simulink model "flightController"  (R2023b)
settings: Solver=ode3  StartTime=0  StopTime=TFinal  FixedStep=Ts  RelTol=1e-3  EnableMultiTasking=on
undefined symbols (not defined in the file): Controller, DiscIntNeverNeededParam, g, PD, PI, PID, Ts, Vehicle
libraries: simulink x7, slpidlib x3, rllib x2, dspstat3 x2, fuzblock x2
(part 1 of 2)
settings Model: Creator=The MathWorks, Inc.  LastModifiedBy=mrkaplan
settings SolverCC: AlgebraicLoopSolver=TrustRegion  MinimalZcImpactIntegration=on
settings DataIOCC: LimitDataPoints=on  SaveFormat=Array  ReturnWorkspaceOutputs=off
settings OptimizationCC: BlockReduction=off  DefaultParameterBehavior=Inlined  BufferReuse=off  PassReuseOutputArgsThreshold=0
settings DebuggingCC: AlgebraicLoopMsg=none  MultiTaskRateTransMsg=warning  ParameterPrecisionLossMsg=none  ParameterTunabilityLossMsg=error  BusObjectLabelMismatch=error  SFUnexpectedBacktrackingDiag=warning  SFNoUnconditionalDefaultTransitionDiag=warning  SFExecutionAtInitializationDiag=none  ArithmeticOperatorsInVariantConditions=warning
settings HardwareCC: ProdBitPerPointer=32  ProdBitPerSizeT=32  ProdBitPerPtrDiffT=32  ProdLargestAtomicInteger=Long  ProdWordSize=32  ProdHWDeviceType=ARM Compatible->ARM 9
settings ModelReferenceCC: EnableRefExpFcnMdlSchedulingChecks=on  ModelReferenceNumInstancesAllowed=Single  PropagateSignalLabelsOutOfModel=off
settings SFSimCC: SimUseLocalCustomCode=off  CustomCodeUndefinedFunction=UseInterfaceOnly
settings RTWCC: GenerateReport=on  RTWUseLocalCustomCode=off  LaunchReport=on
settings CodeAppCC: ForceParamTrailComments=on  MaxIdLength=63  OperatorAnnotations=on  StateflowObjectComments=on  MATLABSourceComments=on
settings GRTTargetCC: TargetLangStandard=C89/C90 (ANSI)
settings ConfigComp: CovMetricSettings=dw  CovSaveCumulativeToWorkspaceVar=on  CovSaveSingleToWorkspaceVar=on  CovExternalEMLEnable=off  CovSFcnEnable=off

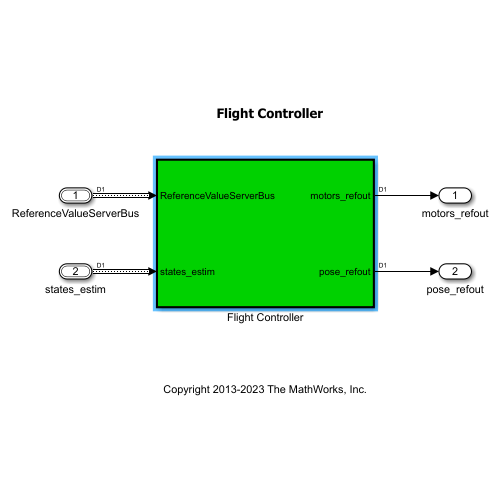
[thumbnail: Simulink's stored preview of the top-level diagram]
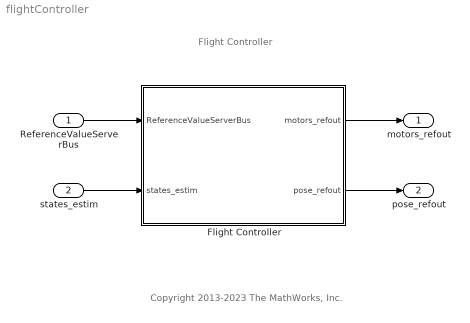
== system flightController ==
  note: Flight Controller
  note: Copyright 2013-2023 The MathWorks, Inc.
  ReferenceValueServerBus : Inport  OutDataTypeStr=Bus: CommandBus  BusOutputAsStruct=on
  states_estim : Inport  Port=2  OutDataTypeStr=Bus: statesEstim_t  BusOutputAsStruct=on
  Flight Controller : Subsystem  TreatAsAtomicUnit=on
  motors_refout : Outport  VectorParamsAs1DForOutWhenUnconnected=off
  pose_refout : Outport  Port=2  VectorParamsAs1DForOutWhenUnconnected=off
  wires:
  ReferenceValueServerBus/1 -> Flight Controller/1(ReferenceValueServerBus)
  states_estim/1 -> Flight Controller/2(states_estim)
  Flight Controller/2(pose_refout) -> pose_refout/1
  Flight Controller/1(motors_refout) -> motors_refout/1

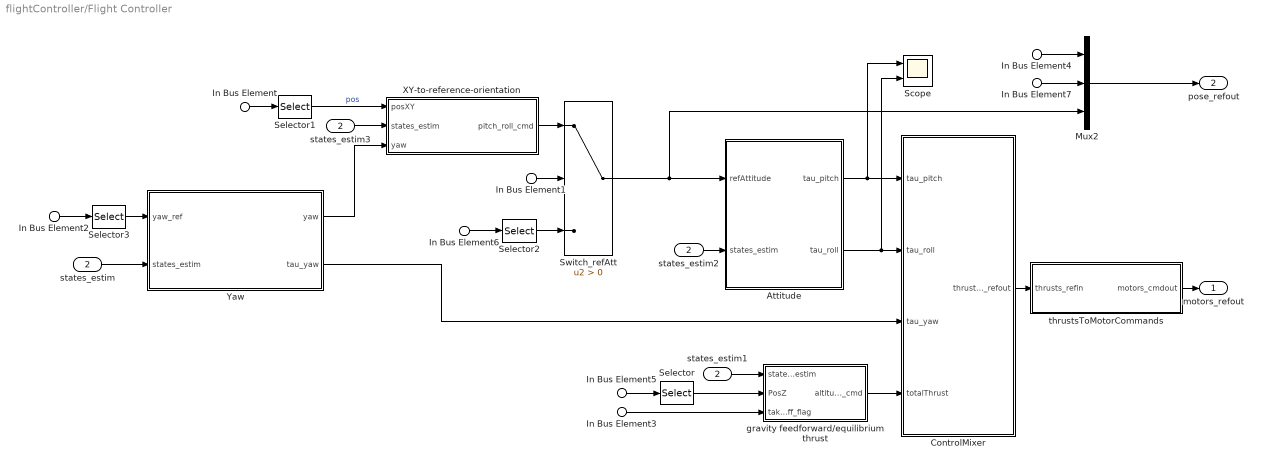
== system flightController/Flight Controller ==
  In Bus Element1 : Inport  PortName=ReferenceValueServerBus  Element=controlModePosVSOrient
  In Bus Element : Inport  PortName=ReferenceValueServerBus  Element=pos_ref
  In Bus Element4 : Inport  PortName=ReferenceValueServerBus  Element=pos_ref
  In Bus Element5 : Inport  PortName=ReferenceValueServerBus  Element=pos_ref
  In Bus Element2 : Inport  PortName=ReferenceValueServerBus  Element=orient_ref
  In Bus Element6 : Inport  PortName=ReferenceValueServerBus  Element=orient_ref
  In Bus Element7 : Inport  PortName=ReferenceValueServerBus  Element=orient_ref
  In Bus Element3 : Inport  PortName=ReferenceValueServerBus  Element=takeoff_flag
  states_estim : Inport  Port=2
  Attitude : Subsystem  Variant=on  VariantControlMode=label  VariantControl=Attitude  LabelModeActiveChoice=RL
  ControlMixer : Subsystem
  Mux2 : Mux  Inputs=3
  Scope : Scope  NumInputPorts=2
  Selector : Selector  InputPortWidth=3  IndexOptions=Index vector (dialog)  Indices=3  OutputSizes=1
  Selector1 : Selector  InputPortWidth=3  IndexOptions=Index vector (dialog)  Indices=[1 2]  OutputSizes=1
  Selector2 : Selector  InputPortWidth=3  IndexOptions=Index vector (dialog)  Indices=[2 3]  OutputSizes=1
  Selector3 : Selector  InputPortWidth=3  IndexOptions=Index vector (dialog)  Indices=1  OutputSizes=1
  Switch_refAtt : Switch  Criteria=u2 > Threshold  SaturateOnIntegerOverflow=off  InputSameDT=off
  XY-to-reference-orientation : Subsystem
  Yaw : Subsystem  Variant=on  VariantControlMode=label  VariantControl=Yaw  LabelModeActiveChoice=PD
  gravity feedforward/equilibrium thrust : Subsystem
  states_estim1 : InportShadow  Port=2
  states_estim2 : InportShadow  Port=2
  states_estim3 : InportShadow  Port=2
  thrustsToMotorCommands : Subsystem
  motors_refout : Outport  VectorParamsAs1DForOutWhenUnconnected=off
  pose_refout : Outport  Port=2  VectorParamsAs1DForOutWhenUnconnected=off
  wires:
  thrustsToMotorCommands/1(motors_cmdout) -> motors_refout/1
  In Bus Element1/1 -> Switch_refAtt/2
  XY-to-reference-orientation/1(pitch_roll_cmd) -> Switch_refAtt/1
  In Bus Element2/1 -> Selector3/1
  In Bus Element/1 -> Selector1/1
  Selector1/1 -> XY-to-reference-orientation/1(posXY)  "pos"
  ControlMixer/1(thrusts_refout) -> thrustsToMotorCommands/1(thrusts_refin)
  In Bus Element3/1 -> gravity feedforward/equilibrium thrust/3(takeoff_flag)
  Switch_refAtt/1 -> Mux2/3, Attitude/1(refAttitude)
  gravity feedforward/equilibrium thrust/1(altitude_cmd) -> ControlMixer/4(totalThrust)
  Mux2/1 -> pose_refout/1
  states_estim1/1 -> gravity feedforward/equilibrium thrust/1(states_estim)
  states_estim3/1 -> XY-to-reference-orientation/2(states_estim)
  In Bus Element4/1 -> Mux2/1
  Selector/1 -> gravity feedforward/equilibrium thrust/2(PosZ)
  In Bus Element5/1 -> Selector/1
  In Bus Element6/1 -> Selector2/1
  Selector2/1 -> Switch_refAtt/3
  In Bus Element7/1 -> Mux2/2
  states_estim2/1 -> Attitude/2(states_estim)
  Attitude/1(tau_pitch) -> Scope/1, ControlMixer/1(tau_pitch)
  Attitude/2(tau_roll) -> Scope/2, ControlMixer/2(tau_roll)
  Selector3/1 -> Yaw/1(yaw_ref)
  states_estim/1 -> Yaw/2(states_estim)
  Yaw/1(yaw) -> XY-to-reference-orientation/3(yaw)
  Yaw/2(tau_yaw) -> ControlMixer/3(tau_yaw)

== system flightController/Flight Controller/Attitude ==
  refAttitude : Inport
  states_estim : Inport  Port=2
  Roll & Pitch PID Controller : Subsystem  VariantControl=PID
  Roll & Pitch RL Agent : Subsystem  VariantControl=RL
  Roll & Pitch RL Based PID Controller : Subsystem  VariantControl=RL Based PID
  tau_pitch : Outport
  tau_roll : Outport  Port=2

== system flightController/Flight Controller/ControlMixer ==
  tau_pitch : Inport
  tau_roll : Inport  Port=2
  tau_yaw : Inport  Port=3
  totalThrust : Inport  Port=4
  Mux2 : Mux
  Product : Product  Multiplication=Matrix(*)  RndMeth=Zero
  TorqueTotalThrustToThrustPerMotor : Constant  Value=Controller.Q2Ts  OutDataTypeStr=single
  thrusts_refout : Outport  VectorParamsAs1DForOutWhenUnconnected=off
  wires:
  Product/1 -> thrusts_refout/1
  tau_roll/1 -> Mux2/4
  tau_pitch/1 -> Mux2/3
  tau_yaw/1 -> Mux2/2
  totalThrust/1 -> Mux2/1
  TorqueTotalThrustToThrustPerMotor/1 -> Product/1
  Mux2/1 -> Product/2

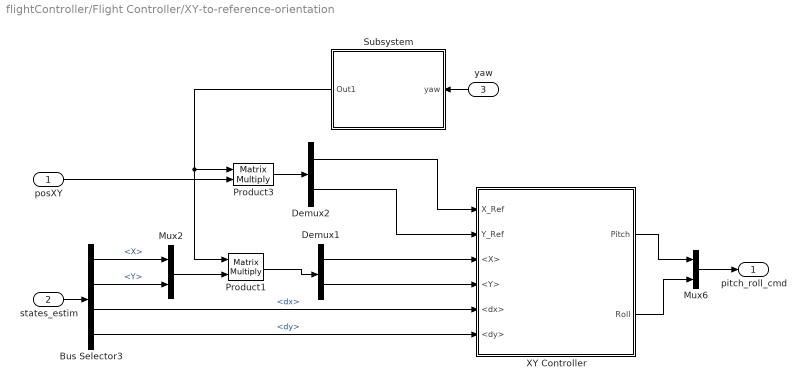
== system flightController/Flight Controller/XY-to-reference-orientation ==
  posXY : Inport
  states_estim : Inport  Port=2
  yaw : Inport  Port=3
  Bus Selector3 : BusSelector  OutputSignals=X,Y,dx,dy
  Demux1 : Demux  Outputs=2
  Demux2 : Demux  Outputs=2
  Mux2 : Mux  Inputs=2
  Mux6 : Mux  Inputs=2
  Product1 : Product  Multiplication=Matrix(*)  OutDataTypeStr=single  RndMeth=Zero
  Product3 : Product  Multiplication=Matrix(*)  OutDataTypeStr=single  RndMeth=Zero
  Subsystem : Subsystem
  "XY Controller " : Subsystem  Variant=on  VariantControlMode=label  VariantControl=Variant2  LabelModeActiveChoice=PD
  pitch_roll_cmd : Outport  VectorParamsAs1DForOutWhenUnconnected=off
  wires:
  Mux6/1 -> pitch_roll_cmd/1
  Demux1/2 -> "XY Controller "/4("<Y> ")
  posXY/1 -> Product3/2
  Demux2/2 -> "XY Controller "/2(Y_Ref)
  Subsystem/1(Out1) -> Product3/1, Product1/1
  Demux2/1 -> "XY Controller "/1(X_Ref)
  states_estim/1 -> Bus Selector3/1
  Demux1/1 -> "XY Controller "/3("<X> ")
  Mux2/1 -> Product1/2
  yaw/1 -> Subsystem/1(yaw)
  Product1/1 -> Demux1/1
  Bus Selector3/3 -> "XY Controller "/5("<dx> ")  "<dx>"
  Bus Selector3/4 -> "XY Controller "/6("<dy> ")  "<dy>"
  Bus Selector3/2 -> Mux2/2  "<Y>"
  Bus Selector3/1 -> Mux2/1  "<X>"
  Product3/1 -> Demux2/1
  "XY Controller "/1(" Pitch") -> Mux6/1
  "XY Controller "/2(" Roll") -> Mux6/2

== system flightController/Flight Controller/Yaw ==
  yaw_ref : Inport
  states_estim : Inport  Port=2
  Yaw PD Controller : Subsystem  VariantControl=PD
  Yaw RL Agent : Subsystem  VariantControl=RL
  yaw : Outport
  tau_yaw : Outport  Port=2

== system flightController/Flight Controller/gravity feedforward//equilibrium thrust ==
  note: ALTITUDE
  states_estim : Inport
  PosZ : Inport  Port=2
  takeoff_flag : Inport  Port=3
  Bus Selector6 : BusSelector  OutputSignals=Z,dz
  SaturationThrust : Saturate  UpperLimit=4*Controller.totalThrustMaxRelative*Controller.motorsThrustPerMotorMax  LowerLimit=-4*Controller.totalThrustMaxRelative*Controller.motorsThrustPerMotorMax  OutDataTypeStr=single
  Sum4 : Sum  Inputs=++|  OutDataTypeStr=single  AccumDataTypeStr=single  SaturateOnIntegerOverflow=on
  TakeoffOrControl_Switch : Switch  Criteria=u2 > Threshold  SaturateOnIntegerOverflow=off  InputSameDT=off
  Z Controller Subsystem : Subsystem  Variant=on  VariantControlMode=label  VariantControl=Variant2  LabelModeActiveChoice=PD
  takeoff_gain : Gain  Gain=Controller.takeoffGain  ParamDataTypeStr=single  OutDataTypeStr=single  SaturateOnIntegerOverflow=on
  w0 : Constant  Value=-g*Vehicle.Airframe.mass  OutDataTypeStr=single  SampleTime=Ts
  altitude_cmd : Outport  VectorParamsAs1DForOutWhenUnconnected=off
  wires:
  Z Controller Subsystem/1(" Altitude") -> TakeoffOrControl_Switch/3
  takeoff_flag/1 -> TakeoffOrControl_Switch/2
  PosZ/1 -> Z Controller Subsystem/1("PosZ ")
  states_estim/1 -> Bus Selector6/1
  takeoff_gain/1 -> TakeoffOrControl_Switch/1
  Sum4/1 -> SaturationThrust/1
  w0/1 -> Sum4/1, takeoff_gain/1
  Bus Selector6/2 -> Z Controller Subsystem/3("<dz> ")  "<dz>"
  SaturationThrust/1 -> altitude_cmd/1
  Bus Selector6/1 -> Z Controller Subsystem/2("<Z> ")  "<Z>"
  TakeoffOrControl_Switch/1 -> Sum4/2

== system flightController/Flight Controller/thrustsToMotorCommands ==
  thrusts_refin : Inport
  MotorDirections : Gain  Gain=[1 -1 1 -1]
  Saturation5 : Saturate  UpperLimit=Vehicle.Motor.maxLimit  LowerLimit=Vehicle.Motor.minLimit
  ThrustToMotorCommand : Gain  Gain=-Vehicle.Motor.thrustToMotorCommand
  motors_cmdout : Outport  VectorParamsAs1DForOutWhenUnconnected=off
  wires:
  Saturation5/1 -> MotorDirections/1
  MotorDirections/1 -> motors_cmdout/1
  ThrustToMotorCommand/1 -> Saturation5/1
  thrusts_refin/1 -> ThrustToMotorCommand/1

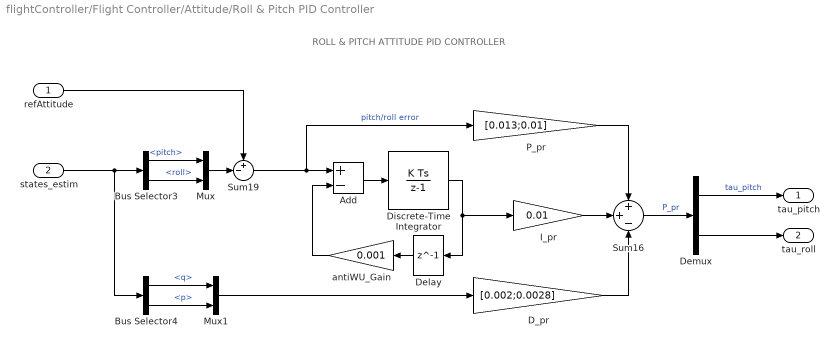
== system flightController/Flight Controller/Attitude/Roll & Pitch PID Controller ==
  note: ROLL & PITCH ATTITUDE PID CONTROLLER
  refAttitude : Inport
  states_estim : Inport  Port=2
  Add : Sum  Inputs=+-
  Bus Selector3 : BusSelector  OutputSignals=pitch,roll
  Bus Selector4 : BusSelector  OutputSignals=q,p
  D_pr : Gain  Gain=[0.002;0.0028]
  Delay : Delay  DelayLength=1  InitialCondition=0
  Demux : Demux  Outputs=2
  Discrete-Time Integrator : DiscreteIntegrator  SampleTime=Ts  LimitOutput=on  UpperSaturationLimit=2  LowerSaturationLimit=-2  ICPrevOutput=DiscIntNeverNeededParam  ICPrevScaledInput=DiscIntNeverNeededParam
  I_pr : Gain  Gain=0.01
  Mux : Mux  Inputs=2
  Mux1 : Mux  Inputs=2
  P_pr : Gain  Gain=[0.013;0.01]
  Sum16 : Sum  Inputs=++-  OutDataTypeStr=single  AccumDataTypeStr=single  SaturateOnIntegerOverflow=on
  Sum19 : Sum  Inputs=+-|
  antiWU_Gain : Gain  Gain=0.001
  tau_pitch : Outport  VectorParamsAs1DForOutWhenUnconnected=off
  tau_roll : Outport  Port=2  VectorParamsAs1DForOutWhenUnconnected=off
  wires:
  Sum16/1 -> Demux/1  "P_pr"
  antiWU_Gain/1 -> Add/2
  Add/1 -> Discrete-Time Integrator/1
  Bus Selector3/1 -> Mux/1  "<pitch>"
  Bus Selector4/1 -> Mux1/1  "<q>"
  P_pr/1 -> Sum16/1
  I_pr/1 -> Sum16/2
  Sum19/1 -> Add/1, P_pr/1  "pitch/roll error"
  Discrete-Time Integrator/1 -> Delay/1, I_pr/1
  Delay/1 -> antiWU_Gain/1
  Demux/1 -> tau_pitch/1  "tau_pitch"
  Demux/2 -> tau_roll/1
  D_pr/1 -> Sum16/3
  states_estim/1 -> Bus Selector3/1, Bus Selector4/1
  refAttitude/1 -> Sum19/1
  Mux/1 -> Sum19/2
  Bus Selector3/2 -> Mux/2  "<roll>"
  Mux1/1 -> D_pr/1
  Bus Selector4/2 -> Mux1/2  "<p>"

== system flightController/Flight Controller/Attitude/Roll & Pitch RL Agent ==
  note: RL BASED ROLL & PITCH ATTITUDE CONTROLLER
  refAttitude : Inport
  states_estim : Inport  Port=2
  Data Type Conversion : DataTypeConversion  OutDataTypeStr=single  SaturateOnIntegerOverflow=off  RndMeth=Floor
  Demux : Demux  Outputs=2
  Display : Display
  RL Agent : rllib/RL Agent  Agent=PPOagentObj  ExternalActionAsInput=off  ProvideLastAction=off  ProvideCumRwd=on  TreatAsDirectFeedthrough=on  UseStrictObservationDataTypes=off
  Saturation : Saturate  UpperLimit=0.005  LowerLimit=-0.005
  Saturation1 : Saturate  UpperLimit=0.005  LowerLimit=-0.005
  Unit Delay : UnitDelay  SampleTime=-1  HasFrameUpgradeWarning=on
  observations : Subsystem
  rewardFunction : Subsystem
      settings: PortSchema="{\"entries\":[{\"content\":{\"sides\":[{\"content\":{\"connectorIds\":[\"In1\",\"In2\"]},\"type\":\"ConnectorPlacement.EquallySpacedRectSide\",\"uuid\":\"a67b2643-6d4e-47da-9384-3a1e9a412811\"},{\"content\":{\"connectorIds\":[\"Out1\",\"Out2\"],\"side\":\"RIGHT\"},\"type\":\"ConnectorPlacement.EquallySpacedRectSide\",\"uuid\":\"5cf99017-b414-4804-a368-110af44f7389\"},{\"content\":{\"connectorIds\":[\"In3\"],\"side\":\"TOP\"},\"type\":\"ConnectorPlacement.EquallySpacedRectSide\",\"uuid\":\"c082dbf4-38c8-469f-94b4-9bfadc9c0830\"}]},\"type\":\"ConnectorPlacement.EquallySpacedConnector\",\"uuid\":\"aea0a46f-4b15-48f6-a1a1-f72f4d47f5c8\"}],\"packageUris\":[\"http://schema.mathworks.com/mf0/Connector/R2020b\"],\"version\":\"1.0\"}"
  tau_pitch : Outport  VectorParamsAs1DForOutWhenUnconnected=off
  tau_roll : Outport  Port=2  VectorParamsAs1DForOutWhenUnconnected=off
  wires:
  rewardFunction/1(Out1) -> RL Agent/2
  refAttitude/1 -> observations/1(refAttitude), rewardFunction/1(In2)
  states_estim/1 -> observations/2(states_estim), rewardFunction/2(In1)
  Demux/2 -> Saturation1/1  "tau_roll"
  Demux/1 -> Saturation/1  "tau_pitch"
  RL Agent/1 -> Unit Delay/1, Data Type Conversion/1
  Data Type Conversion/1 -> Demux/1
  observations/1(Out1) -> RL Agent/1
  rewardFunction/2(Out2) -> RL Agent/3
  Saturation/1 -> tau_pitch/1
  Saturation1/1 -> tau_roll/1
  RL Agent/2 -> Display/1
  Unit Delay/1 -> rewardFunction/3(In3)

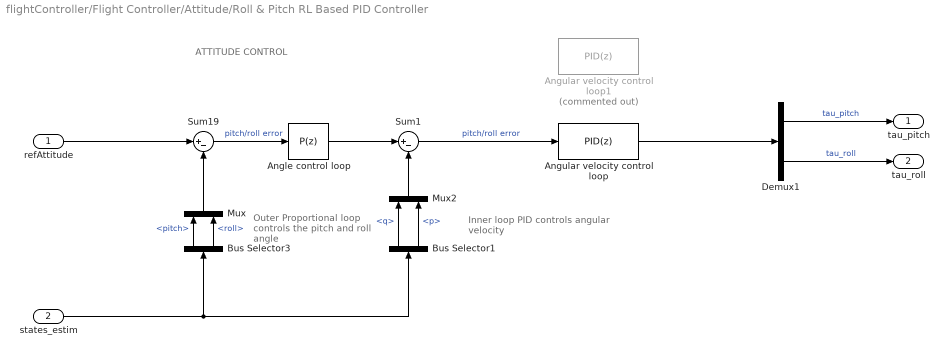
== system flightController/Flight Controller/Attitude/Roll & Pitch RL Based PID Controller ==
  note: ATTITUDE CONTROL
  note: Inner loop PID
      | controls angular velocity
  note: Outer Proportional loop
      | controls the pitch and roll angle
  refAttitude : Inport
  states_estim : Inport  Port=2
  Angle control loop : slpidlib/PID Controller  Controller=P  Form=Parallel  TimeDomain=Discrete-time  UseExternalTs=off  SampleTime=Ts  IntegratorMethod=Forward Euler  FilterMethod=Forward Euler  ControllerParametersSource=internal  P=4  I=1  UseKiTs=off  D=0  N=100  UseFilter=on  TunerSelectOption=Transfer Function Based (PID Tuner App)  InitialConditionSource=internal  InitialConditionForIntegrator=0  InitialConditionForFilter=0  DifferentiatorICPrevScaledInput=0  ExternalReset=none  TrackingMode=off  Kt=1  LimitOutput=off  SatLimitsSource=internal  UpperSaturationLimit=inf  LowerSaturationLimit=-inf  LinearizeAsGain=on  AntiWindupMode=none  Kb=1  LimitIntegrator=off  UpperIntegratorSaturationLimit=inf  LowerIntegratorSaturationLimit=-inf  POutMin=[]  POutMax=[]  IOutMin=[]  IOutMax=[]  DOutMin=[]  DOutMax=[]  NOutMin=[]  NOutMax=[]  SumOutMin=[]  SumOutMax=[]  SaturationOutMin=[]  SaturationOutMax=[]  PParamMin=[]  PParamMax=[]  IParamMin=[]  IParamMax=[]  DParamMin=[]  DParamMax=[]  NParamMin=[]  NParamMax=[]  KbParamMin=[]  KbParamMax=[]  KtParamMin=[]  KtParamMax=[]  KbOutMin=[]  KbOutMax=[]  KtOutMin=[]  KtOutMax=[]  IntegratorOutMin=[]  IntegratorOutMax=[]  FilterOutMin=[]  FilterOutMax=[]  SumI1OutMin=[]  SumI1OutMax=[]  SumI2OutMin=[]  SumI2OutMax=[]  SumI3OutMin=[]  SumI3OutMax=[]  SumI4OutMin=[]  SumI4OutMax=[]  SumDOutMin=[]  SumDOutMax=[]  DifferentiatorOutMin=[]  DifferentiatorOutMax=[]  FilterDiffOutCoefMin=[]  FilterDiffOutCoefMax=[]  ReciprocalOutMin=[]  ReciprocalOutMax=[]  SumDenOutMin=[]  SumDenOutMax=[]  SumNumOutMin=[]  SumNumOutMax=[]  DivideOutMin=[]  DivideOutMax=[]  UdiffTsProdOutMin=[]  UdiffTsProdOutMax=[]  NTsProdOutMin=[]  NTsProdOutMax=[]  UintegralTsProdOutMin=[]  UintegralTsProdOutMax=[]  UngainTsProdOutMin=[]  UngainTsProdOutMax=[]  ClampingZeroOutDataTypeStr=Inherit: Inherit via back propagation  ClampingZeroOutMin=[]  ClampingZeroOutMax=[]  FilterDenConstantOutDataTypeStr=Inherit: Inherit via back propagation  FilterDenConstantOutMin=[]  FilterDenConstantOutMax=[]  PCopyOutDataTypeStr=Inherit: Inherit via back propagation  PCopyOutMin=[]  PCopyOutMax=[]  NCopyOutDataTypeStr=Inherit: Inherit via back propagation  NCopyOutMin=[]  NCopyOutMax=[]  IntegratorContinuousStateAttributes=''  IntegratorStateMustResolveToSignalObject=off  IntegratorRTWStateStorageClass=Auto  FilterContinuousStateAttributes=''  FilterStateMustResolveToSignalObject=off  FilterRTWStateStorageClass=Auto  ParallelPVariant=InternalParameters  IdealPVariant=Disabled  IVariant=Disabled  DVariant=Disabled  IntegratorVariant=Disabled  SatVariant=Disabled  AWVariant=Disabled  PCopyVariant=Disabled  TRVariant=Disabled  FdbkBlocksVariant=Forward  IdealPFdbkVariant=Disabled  SatFdbkVariant=Disabled  DerivativeFilterVariant=Disabled  NVariant=Disabled  NCopyVariant=Disabled_SignalSpec  FilterICVariant=Disabled  IntegratorICVariant=Disabled  ExternalResetVariant=Disabled  TRSumVariant=Passthrough  SumFdbkVariant=Disabled  SumVariant=Passthrough_P  TsampFilterVariant=InternalTs  TsampNgainVariant=Passthrough  TsampIntegralVariant=Disabled_SignalSpec  ExternalSaturationOutDataTypeStr=Inherit: Same as second input
  Angular velocity control loop : slpidlib/PID Controller  Controller=PID  Form=Parallel  TimeDomain=Discrete-time  UseExternalTs=off  SampleTime=Ts  IntegratorMethod=Forward Euler  FilterMethod=Forward Euler  ControllerParametersSource=internal  P=0.003*[0.1 0.08]  I=2*0.003*[1 0.81]  UseKiTs=off  D=0.003/25*[1 0.81]  N=70*[1 1]  UseFilter=on  TunerSelectOption=Transfer Function Based (PID Tuner App)  InitialConditionSource=internal  InitialConditionForIntegrator=0  InitialConditionForFilter=0  DifferentiatorICPrevScaledInput=0  ExternalReset=none  TrackingMode=off  Kt=1  LimitOutput=on  SatLimitsSource=internal  UpperSaturationLimit=0.02  LowerSaturationLimit=-0.02  LinearizeAsGain=on  AntiWindupMode=clamping  Kb=1  LimitIntegrator=off  UpperIntegratorSaturationLimit=inf  LowerIntegratorSaturationLimit=-inf  POutMin=[]  POutMax=[]  IOutMin=[]  IOutMax=[]  DOutMin=[]  DOutMax=[]  NOutMin=[]  NOutMax=[]  SumOutMin=[]  SumOutMax=[]  SaturationOutMin=[]  SaturationOutMax=[]  PParamMin=[]  PParamMax=[]  IParamMin=[]  IParamMax=[]  DParamMin=[]  DParamMax=[]  NParamMin=[]  NParamMax=[]  KbParamMin=[]  KbParamMax=[]  KtParamMin=[]  KtParamMax=[]  KbOutMin=[]  KbOutMax=[]  KtOutMin=[]  KtOutMax=[]  IntegratorOutMin=[]  IntegratorOutMax=[]  FilterOutMin=[]  FilterOutMax=[]  SumI1OutMin=[]  SumI1OutMax=[]  SumI2OutMin=[]  SumI2OutMax=[]  SumI3OutMin=[]  SumI3OutMax=[]  SumI4OutMin=[]  SumI4OutMax=[]  SumDOutMin=[]  SumDOutMax=[]  DifferentiatorOutMin=[]  DifferentiatorOutMax=[]  FilterDiffOutCoefMin=[]  FilterDiffOutCoefMax=[]  ReciprocalOutMin=[]  ReciprocalOutMax=[]  SumDenOutMin=[]  SumDenOutMax=[]  SumNumOutMin=[]  SumNumOutMax=[]  DivideOutMin=[]  DivideOutMax=[]  UdiffTsProdOutMin=[]  UdiffTsProdOutMax=[]  NTsProdOutMin=[]  NTsProdOutMax=[]  UintegralTsProdOutMin=[]  UintegralTsProdOutMax=[]  UngainTsProdOutMin=[]  UngainTsProdOutMax=[]  ClampingZeroOutDataTypeStr=Inherit: Inherit via back propagation  ClampingZeroOutMin=[]  ClampingZeroOutMax=[]  FilterDenConstantOutDataTypeStr=Inherit: Inherit via back propagation  FilterDenConstantOutMin=[]  FilterDenConstantOutMax=[]  PCopyOutDataTypeStr=Inherit: Inherit via back propagation  PCopyOutMin=[]  PCopyOutMax=[]  NCopyOutDataTypeStr=Inherit: Inherit via back propagation  NCopyOutMin=[]  NCopyOutMax=[]  IntegratorContinuousStateAttributes=''  IntegratorStateMustResolveToSignalObject=off  IntegratorRTWStateStorageClass=Auto  FilterContinuousStateAttributes=''  FilterStateMustResolveToSignalObject=off  FilterRTWStateStorageClass=Auto  ParallelPVariant=InternalParameters  IdealPVariant=Disabled  IVariant=InternalParameters  DVariant=InternalParameters  IntegratorVariant=Discrete  SatVariant=Enabled  AWVariant=DiscClampingParallel  PCopyVariant=Disabled  TRVariant=Disabled  FdbkBlocksVariant=Forward  IdealPFdbkVariant=Disabled  SatFdbkVariant=Disabled  DerivativeFilterVariant=ForwardEulerFilter  NVariant=InternalParameters  NCopyVariant=Disabled  FilterICVariant=InternalICsFilter  IntegratorICVariant=InternalICs  ExternalResetVariant=Disabled  TRSumVariant=Passthrough  SumFdbkVariant=Disabled  SumVariant=Sum_PID  TsampFilterVariant=InternalTs  TsampNgainVariant=Passthrough  TsampIntegralVariant=Disabled_SignalSpec  ExternalSaturationOutDataTypeStr=Inherit: Same as second input
  Angular velocity control loop1 : slpidlib/PID Controller  Commented=on  Controller=PID  Form=Parallel  TimeDomain=Discrete-time  UseExternalTs=off  SampleTime=Ts  IntegratorMethod=Forward Euler  FilterMethod=Forward Euler  ControllerParametersSource=internal  P=0.003*[1 0.81]  I=2*0.003*[1 0.81]  UseKiTs=off  D=0.003/25*[1 0.81]  N=70*[1 1]  UseFilter=on  TunerSelectOption=Transfer Function Based (PID Tuner App)  InitialConditionSource=internal  InitialConditionForIntegrator=0  InitialConditionForFilter=0  DifferentiatorICPrevScaledInput=0  ExternalReset=none  TrackingMode=off  Kt=1  LimitOutput=on  SatLimitsSource=internal  UpperSaturationLimit=0.02  LowerSaturationLimit=-0.02  LinearizeAsGain=on  AntiWindupMode=clamping  Kb=1  LimitIntegrator=off  UpperIntegratorSaturationLimit=inf  LowerIntegratorSaturationLimit=-inf  POutMin=[]  POutMax=[]  IOutMin=[]  IOutMax=[]  DOutMin=[]  DOutMax=[]  NOutMin=[]  NOutMax=[]  SumOutMin=[]  SumOutMax=[]  SaturationOutMin=[]  SaturationOutMax=[]  PParamMin=[]  PParamMax=[]  IParamMin=[]  IParamMax=[]  DParamMin=[]  DParamMax=[]  NParamMin=[]  NParamMax=[]  KbParamMin=[]  KbParamMax=[]  KtParamMin=[]  KtParamMax=[]  KbOutMin=[]  KbOutMax=[]  KtOutMin=[]  KtOutMax=[]  IntegratorOutMin=[]  IntegratorOutMax=[]  FilterOutMin=[]  FilterOutMax=[]  SumI1OutMin=[]  SumI1OutMax=[]  SumI2OutMin=[]  SumI2OutMax=[]  SumI3OutMin=[]  SumI3OutMax=[]  SumI4OutMin=[]  SumI4OutMax=[]  SumDOutMin=[]  SumDOutMax=[]  DifferentiatorOutMin=[]  DifferentiatorOutMax=[]  FilterDiffOutCoefMin=[]  FilterDiffOutCoefMax=[]  ReciprocalOutMin=[]  ReciprocalOutMax=[]  SumDenOutMin=[]  SumDenOutMax=[]  SumNumOutMin=[]  SumNumOutMax=[]  DivideOutMin=[]  DivideOutMax=[]  UdiffTsProdOutMin=[]  UdiffTsProdOutMax=[]  NTsProdOutMin=[]  NTsProdOutMax=[]  UintegralTsProdOutMin=[]  UintegralTsProdOutMax=[]  UngainTsProdOutMin=[]  UngainTsProdOutMax=[]  ClampingZeroOutDataTypeStr=Inherit: Inherit via back propagation  ClampingZeroOutMin=[]  ClampingZeroOutMax=[]  FilterDenConstantOutDataTypeStr=Inherit: Inherit via back propagation  FilterDenConstantOutMin=[]  FilterDenConstantOutMax=[]  PCopyOutDataTypeStr=Inherit: Inherit via back propagation  PCopyOutMin=[]  PCopyOutMax=[]  NCopyOutDataTypeStr=Inherit: Inherit via back propagation  NCopyOutMin=[]  NCopyOutMax=[]  IntegratorContinuousStateAttributes=''  IntegratorStateMustResolveToSignalObject=off  IntegratorRTWStateStorageClass=Auto  FilterContinuousStateAttributes=''  FilterStateMustResolveToSignalObject=off  FilterRTWStateStorageClass=Auto  ParallelPVariant=InternalParameters  IdealPVariant=Disabled  IVariant=InternalParameters  DVariant=InternalParameters  IntegratorVariant=Discrete  SatVariant=Enabled  AWVariant=DiscClampingParallel  PCopyVariant=Disabled  TRVariant=Disabled  FdbkBlocksVariant=Forward  IdealPFdbkVariant=Disabled  SatFdbkVariant=Disabled  DerivativeFilterVariant=ForwardEulerFilter  NVariant=InternalParameters  NCopyVariant=Disabled  FilterICVariant=InternalICsFilter  IntegratorICVariant=InternalICs  ExternalResetVariant=Disabled  TRSumVariant=Passthrough  SumFdbkVariant=Disabled  SumVariant=Sum_PID  TsampFilterVariant=InternalTs  TsampNgainVariant=Passthrough  TsampIntegralVariant=Disabled_SignalSpec  ExternalSaturationOutDataTypeStr=Inherit: Same as second input
  Bus Selector1 : BusSelector  OutputSignals=q,p
  Bus Selector3 : BusSelector  OutputSignals=pitch,roll
  Demux1 : Demux  Outputs=2
  Mux : Mux  Inputs=2
  Mux2 : Mux  Inputs=2
  Sum1 : Sum  Inputs=|+-
  Sum19 : Sum  Inputs=|+-
  tau_pitch : Outport  VectorParamsAs1DForOutWhenUnconnected=off
  tau_roll : Outport  Port=2  VectorParamsAs1DForOutWhenUnconnected=off
  wires:
  Bus Selector1/2 -> Mux2/2  "<p>"
  states_estim/1 -> Bus Selector1/1, Bus Selector3/1
  Angular velocity control loop/1 -> Demux1/1
  Bus Selector1/1 -> Mux2/1  "<q>"
  Sum1/1 -> Angular velocity control loop/1  "pitch/roll error"
  Angle control loop/1 -> Sum1/1
  Demux1/2 -> tau_roll/1  "tau_roll"
  Demux1/1 -> tau_pitch/1  "tau_pitch"
  Bus Selector3/2 -> Mux/2  "<roll>"
  Sum19/1 -> Angle control loop/1  "pitch/roll error"
  refAttitude/1 -> Sum19/1
  Bus Selector3/1 -> Mux/1  "<pitch>"
  Mux/1 -> Sum19/2
  Mux2/1 -> Sum1/2

== system flightController/Flight Controller/XY-to-reference-orientation/Subsystem ==
  yaw : Inport
  Gain2 : Gain  Gain=-1
  Matrix Concatenate1 : Concatenate  Mode=Multidimensional array  ConcatenateDimension=2
  Trigonometric Function1 : Trigonometry  Operator=sincos
  Vector Concatenate2 : Concatenate
  Vector Concatenate3 : Concatenate
  Out1 : Outport  VectorParamsAs1DForOutWhenUnconnected=off
  wires:
  Trigonometric Function1/2 -> Vector Concatenate3/2, Vector Concatenate2/1
  Vector Concatenate3/1 -> Matrix Concatenate1/2
  yaw/1 -> Trigonometric Function1/1
  Gain2/1 -> Vector Concatenate2/2
  Vector Concatenate2/1 -> Matrix Concatenate1/1
  Trigonometric Function1/1 -> Gain2/1, Vector Concatenate3/1
  Matrix Concatenate1/1 -> Out1/1

== system flightController/Flight Controller/XY-to-reference-orientation/XY Controller  ==
  X_Ref : Inport
  Y_Ref : Inport  Port=2
  "<X> " : Inport  Port=3
  "<Y> " : Inport  Port=4
  "<dx> " : Inport  Port=5
  "<dy> " : Inport  Port=6
  "(Fuzzy PI) - PD Controller " : Subsystem  VariantControl=Fuzzy PI - PD  mask{Kc=-0.238682, Td=0.682112, b=1, K0=1.7, Ke=1, Kd=0.9}
      mask prompts: Kc "Kc (Proportional)"; Td "Td (Derivative)"; b "b (Setpoint weight)"
      mask help: Example of a Fuzzy PI - PD Controller subsystem. Controller parameters for XY to reference orientation
      mask init:
      | block = find_system(gcb,...
      |           'LookUnderMasks','on',...
      |           'FollowLinks','on','Name','In2');
      mask DialogControl ParameterGroupVar Prompt: PD internal controller
      mask DialogControl Container3 Prompt: Fuzzy PI external controller
  "PD Controller " : Subsystem  VariantControl=PD  mask{Kc=-0.24, Td=0.1/0.24, b=1}
      mask prompts: Kc "Kc (Proportional)"; Td "Td (Derivative)"; b "b (Setpoint weight)"
      mask help: Example of a 2-DOF PD Controller subsystem. Controller parameters for XY to reference orientation
      mask init:
      | block = find_system(gcb,...
      |           'LookUnderMasks','on',...
      |           'FollowLinks','on','Name','In2');
  "PI-PD Controller " : Subsystem  VariantControl=PI-PD  mask{Kc=-0.24, Td=0.1/0.24, b=1, Kp=0.25, Ki=0.5, Kf=0.0}
      mask prompts: Kc "Kc (Proportional)"; Td "Td (Derivative)"; b "b (Setpoint weight)"; Kp "Kp (Proportional Gain)"; Ki "Ki (Integral Gain)"; Kf "Kf (Feedforward Gain)"
      mask help: Example of a 2-DOF PI-PD Controller subsystem. Controller parameters for XY to reference orientation
      mask init:
      | block = find_system(gcb,...
      |           'LookUnderMasks','on',...
      |           'FollowLinks','on','Name','In2');
      mask DialogControl ParameterGroupVar Prompt: PD internal controller
      mask DialogControl Container3 Prompt: PI external controller
      mask DialogControl Container4 Prompt: Feedforward Gain
  "PID-PD Controller " : Subsystem  VariantControl=PID-PD  mask{Kc=-0.238682, Td=0.682112, b=1, Kp=0.25, Ki=0.5, Kd=0.0, Kf=0.0}
      mask prompts: Kc "Kc (Proportional)"; Td "Td (Derivative)"; b "b (Setpoint weight)"; Kp "Kp (Proportional Gain)"; Ki "Ki (Integral Gain)"; Kd "Kd (Derivative Gain)"; Kf "Kf (Feedforward Gain)"
      mask help: Example of a 2-DOF PID-PD Controller subsystem. Controller parameters for XY to reference orientation
      mask init:
      | block = find_system(gcb,...
      |           'LookUnderMasks','on',...
      |           'FollowLinks','on','Name','In2');
      mask DialogControl ParameterGroupVar Prompt: PD internal controller
      mask DialogControl Container3 Prompt: PID external controller
      mask DialogControl Container4 Prompt: Feedforward Gain
  " Pitch" : Outport  VectorParamsAs1DForOutWhenUnconnected=off
  " Roll" : Outport  Port=2  VectorParamsAs1DForOutWhenUnconnected=off

== system flightController/Flight Controller/Yaw/Yaw PD Controller ==
  note: YAW ATTITUDE PD CONTROLLER
  yaw_ref : Inport
  states_estim : Inport  Port=2
  Bus Selector5 : BusSelector  OutputSignals=yaw,r
  D_yaw : Gain  Gain=0.3*0.004
  P_yaw : Gain  Gain=0.004  ParamDataTypeStr=single  OutDataTypeStr=single
  Sum1 : Sum  Inputs=+-|  OutDataTypeStr=single  AccumDataTypeStr=single  SaturateOnIntegerOverflow=on
  Sum2 : Sum  Inputs=|+-
  yaw : Outport  VectorParamsAs1DForOutWhenUnconnected=off
  tau_yaw : Outport  Port=2  VectorParamsAs1DForOutWhenUnconnected=off
  wires:
  D_yaw/1 -> Sum2/2
  P_yaw/1 -> Sum2/1
  Bus Selector5/2 -> D_yaw/1  "<r>"
  Sum1/1 -> P_yaw/1
  states_estim/1 -> Bus Selector5/1
  Sum2/1 -> tau_yaw/1
  Bus Selector5/1 -> yaw/1, Sum1/2  "<yaw>"
  yaw_ref/1 -> Sum1/1

== system flightController/Flight Controller/Yaw/Yaw RL Agent ==
  note: RL BASED YAW ATTITUDE CONTROLLER
  yaw_ref : Inport
  states_estim : Inport  Port=2
  Data Type Conversion : DataTypeConversion  OutDataTypeStr=single  SaturateOnIntegerOverflow=off  RndMeth=Floor
  RL Agent : rllib/RL Agent  Agent=PPOagent2Obj  ExternalActionAsInput=off  ProvideLastAction=off  ProvideCumRwd=off  TreatAsDirectFeedthrough=on  UseStrictObservationDataTypes=off
  observations : Subsystem
      settings: PortSchema="{\"entries\":[{\"content\":{\"sides\":[{\"content\":{\"connectorIds\":[\"In1\"]},\"type\":\"ConnectorPlacement.EquallySpacedRectSide\",\"uuid\":\"a3b67cbb-e476-4be2-be7c-7eea36da381b\"},{\"content\":{\"connectorIds\":[\"Out1\"],\"side\":\"RIGHT\"},\"type\":\"ConnectorPlacement.EquallySpacedRectSide\",\"uuid\":\"9cf72cce-49c7-479d-af00-70c0385ccd4a\"},{\"content\":{\"connectorIds\":[\"Out2\"],\"side\":\"TOP\"},\"type\":\"ConnectorPlacement.EquallySpacedRectSide\",\"uuid\":\"9ba7e01e-3a67-4c70-88ca-ae7166fdaec1\"}]},\"type\":\"ConnectorPlacement.EquallySpacedConnector\",\"uuid\":\"bb1b65ec-6aa1-4e64-ae81-1263ce455c6c\"}],\"packageUris\":[\"http://schema.mathworks.com/mf0/Connector/R2020b\"],\"version\":\"1.0\"}"
  rewardFunction : Subsystem
  yaw : Outport  VectorParamsAs1DForOutWhenUnconnected=off
  tau_yaw : Outport  Port=2  VectorParamsAs1DForOutWhenUnconnected=off
  wires:
  Data Type Conversion/1 -> tau_yaw/1
  RL Agent/1 -> Data Type Conversion/1
  rewardFunction/2(Out2) -> RL Agent/3
  observations/1(Out1) -> RL Agent/1
  yaw_ref/1 -> rewardFunction/1(yaw_ref)
  states_estim/1 -> observations/1(In1), rewardFunction/2(states_estim)
  rewardFunction/1(Out1) -> RL Agent/2
  observations/2(yaw) -> yaw/1

== system flightController/Flight Controller/gravity feedforward//equilibrium thrust/Z Controller Subsystem ==
  "PosZ " : Inport
  "<Z> " : Inport  Port=2
  "<dz> " : Inport  Port=3
  "PD Controller " : Subsystem  VariantControl=PD  mask{Kc=1.465, Td=0.273, b=1}
      mask prompts: Kc "Kc (Proportional)"; Td "Td (Derivative)"; b "b (Setpoint weight)"
      mask help: Example of a 2-DOF PD Controller subsystem. Controller parameters for Z (Altitude).
      mask init:
      | block = find_system(gcb,...
      |           'LookUnderMasks','on',...
      |           'FollowLinks','on','Name','In2');
  "PI-PD Controller " : Subsystem  VariantControl=PI-PD  mask{Kc=1.465, Td=0.273, b=1, Kp=0.12748, Ki=0.0713}
      mask prompts: Kc "Kc (Proportional)"; Td "Td (Derivative)"; b "b (Setpoint weight)"; Kp "Kp (Proportional Gain)"; Ki "Ki (Integral Gain)"
      mask help: Example of a 2-DOF PI-PD Controller subsystem. Controller parameters for Z (Altitude).
      mask init:
      | block = find_system(gcb,...
      |           'LookUnderMasks','on',...
      |           'FollowLinks','on','Name','In2');
      mask DialogControl ParameterGroupVar Prompt: PD Internal Controller Parameters
      mask DialogControl Container3 Prompt: PI External Controller Parameters
  " Altitude" : Outport  VectorParamsAs1DForOutWhenUnconnected=off

== system flightController/Flight Controller/Attitude/Roll & Pitch RL Agent/observations ==
  refAttitude : Inport
  states_estim : Inport  Port=2
  Bus Selector : BusSelector  OutputSignals=q,p
  Bus Selector1 : BusSelector  OutputSignals=pitch,roll
  Demux : Demux  Outputs=2
  Discrete-Time Integrator : DiscreteIntegrator  SampleTime=Ts  ICPrevOutput=DiscIntNeverNeededParam  ICPrevScaledInput=DiscIntNeverNeededParam
  Discrete-Time Integrator1 : DiscreteIntegrator  SampleTime=Ts  ICPrevOutput=DiscIntNeverNeededParam  ICPrevScaledInput=DiscIntNeverNeededParam
  Mux : Mux  Inputs=6
  Sum : Sum  Inputs=|+-
  Sum1 : Sum  Inputs=|+-
  Out1 : Outport
  wires:
  states_estim/1 -> Bus Selector1/1, Bus Selector/1
  Mux/1 -> Out1/1
  refAttitude/1 -> Demux/1
  Demux/1 -> Sum/1  "pitch_ref"
  Demux/2 -> Sum1/1  "roll_ref"
  Bus Selector1/1 -> Sum/2  "<pitch>"
  Bus Selector1/2 -> Sum1/2  "<roll>"
  Sum/1 -> Discrete-Time Integrator/1, Mux/1
  Discrete-Time Integrator/1 -> Mux/2
  Sum1/1 -> Discrete-Time Integrator1/1, Mux/3
  Discrete-Time Integrator1/1 -> Mux/4
  Bus Selector/1 -> Mux/5  "<q>"
  Bus Selector/2 -> Mux/6  "<p>"

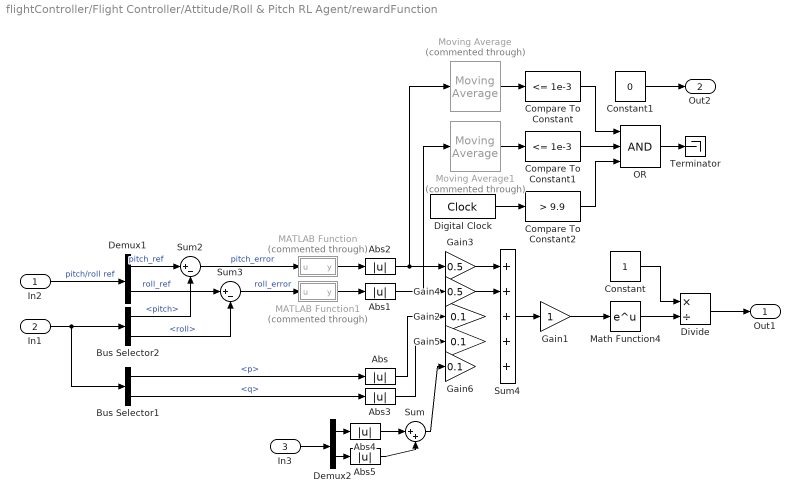
== system flightController/Flight Controller/Attitude/Roll & Pitch RL Agent/rewardFunction ==
  In2 : Inport
  In1 : Inport  Port=2
  In3 : Inport  Port=3
  Abs{,1..5} (6 alike) : Abs  SaturateOnIntegerOverflow=off
  Bus Selector1 : BusSelector  OutputSignals=p,q
  Bus Selector2 : BusSelector  OutputSignals=pitch,roll
  Compare To Constant : simulink/Logic and Bit Operations/Compare To Constant  relop=<=  const=1e-3  OutDataTypeStr=boolean
  Compare To Constant1 : simulink/Logic and Bit Operations/Compare To Constant  relop=<=  const=1e-3  OutDataTypeStr=boolean
  Compare To Constant2 : simulink/Logic and Bit Operations/Compare To Constant  relop=>  const=9.9  OutDataTypeStr=boolean
  Constant : Constant  SampleTime=Ts
  Constant1 : Constant  Value=0  SampleTime=Ts
  Demux1 : Demux  Outputs=2
  Demux2 : Demux  Outputs=2
  Digital Clock : DigitalClock  SampleTime=Ts
  Divide : Product  Inputs=*/
  Gain1 : Gain  OutDataTypeStr=single
  Gain2 : Gain  Gain=0.1
  Gain3 : Gain  Gain=0.5
  Gain4 : Gain  Gain=0.5
  Gain5 : Gain  Gain=0.1
  Gain6 : Gain  Gain=0.1
  MATLAB Function : MATLAB Function  Commented=through  TreatAsAtomicUnit=on
  MATLAB Function1 : MATLAB Function  Commented=through  TreatAsAtomicUnit=on
  Math Function4 : Math
  Moving Average : dspstat3/Moving Average  Commented=through  Method=Sliding window  ForgettingFactorPort=off  SpecifyWindowLength=on  WindowLength=200  OverlapLength=199  AllowArbitraryInputLength=off  ForgettingFactor=0.9  SimulateUsing=Code generation
  Moving Average1 : dspstat3/Moving Average  Commented=through  Method=Sliding window  ForgettingFactorPort=off  SpecifyWindowLength=on  WindowLength=200  OverlapLength=199  AllowArbitraryInputLength=off  ForgettingFactor=0.9  SimulateUsing=Code generation
  OR : Logic  Inputs=3  AllPortsSameDT=off  OutDataTypeStr=boolean
  Sum : Sum  Inputs=|++
  Sum2 : Sum  Inputs=|+-
  Sum3 : Sum  Inputs=|+-
  Sum4 : Sum  Inputs=+++++
  Terminator : Terminator
  Out1 : Outport
  Out2 : Outport  Port=2
  wires:
  In2/1 -> Demux1/1  "pitch/roll ref"
  In1/1 -> Bus Selector1/1, Bus Selector2/1
  Demux1/1 -> Sum2/1  "pitch_ref"
  Demux1/2 -> Sum3/1  "roll_ref"
  Bus Selector2/1 -> Sum2/2  "<pitch>"
  Bus Selector2/2 -> Sum3/2  "<roll>"
  Sum2/1 -> MATLAB Function/1(u)  "pitch_error"
  Sum3/1 -> MATLAB Function1/1(u)  "roll_error"
  Abs2/1 -> Moving Average/1, Gain3/1
  Abs1/1 -> Gain4/1, Moving Average1/1
  Sum4/1 -> Gain1/1
  Gain3/1 -> Sum4/1
  Gain4/1 -> Sum4/2
  Compare To Constant/1 -> OR/1
  Compare To Constant1/1 -> OR/2
  Digital Clock/1 -> Compare To Constant2/1
  Compare To Constant2/1 -> OR/3
  MATLAB Function1/1(y) -> Abs1/1
  MATLAB Function/1(y) -> Abs2/1
  Moving Average/1 -> Compare To Constant/1
  Moving Average1/1 -> Compare To Constant1/1
  Bus Selector1/1 -> Abs/1  "<p>"
  Bus Selector1/2 -> Abs3/1  "<q>"
  Abs/1 -> Gain2/1
  Abs3/1 -> Gain5/1
  In3/1 -> Demux2/1
  Sum/1 -> Gain6/1
  Demux2/1 -> Abs4/1
  Demux2/2 -> Abs5/1
  Abs4/1 -> Sum/1
  Abs5/1 -> Sum/2
  Math Function4/1 -> Divide/2
  Constant/1 -> Divide/1
  Constant1/1 -> Out2/1
  OR/1 -> Terminator/1
  Gain1/1 -> Math Function4/1
  Divide/1 -> Out1/1

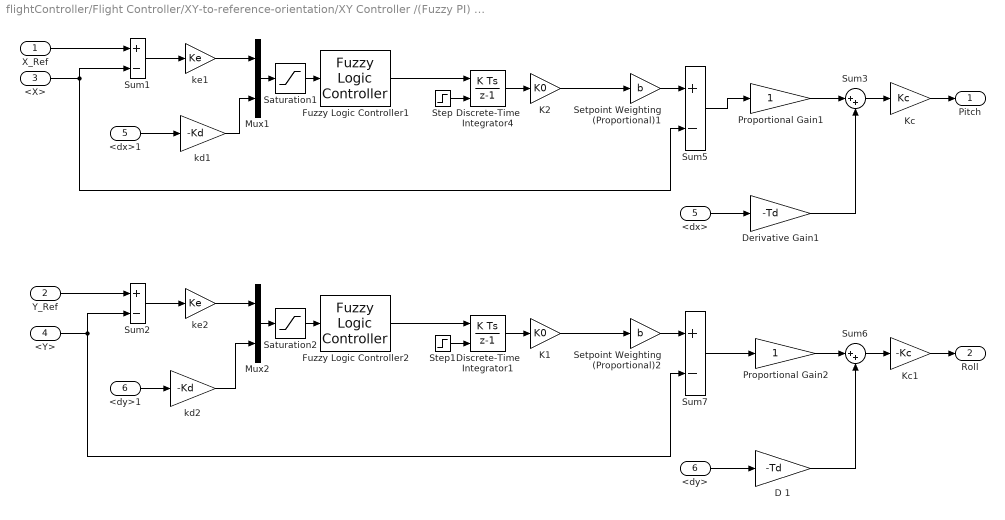
== system flightController/Flight Controller/XY-to-reference-orientation/XY Controller /(Fuzzy PI) - PD Controller  ==
  X_Ref : Inport
  Y_Ref : Inport  Port=2
  <X> : Inport  Port=3
  <Y> : Inport  Port=4
  <dx> : Inport  Port=5
  <dy> : Inport  Port=6
  <dx>1 : InportShadow  Port=5
  <dy>1 : InportShadow  Port=6
  D 1 : Gain  Gain=-Td
  Derivative Gain1 : Gain  DisableCoverage=on  Gain=-Td
  Discrete-Time Integrator1 : DiscreteIntegrator  ExternalReset=falling  SampleTime=Ts  ICPrevOutput=DiscIntNeverNeededParam  ICPrevScaledInput=DiscIntNeverNeededParam
  Discrete-Time Integrator4 : DiscreteIntegrator  ExternalReset=falling  SampleTime=Ts  ICPrevOutput=DiscIntNeverNeededParam  ICPrevScaledInput=DiscIntNeverNeededParam
  Fuzzy Logic Controller1 : fuzblock/Fuzzy Logic  Controller  FIS='Untitled2.fis'  OutputSampleNumber=101  DataType=double  FuzzifiedInputs=off  RuleFiringStrengths=off  RuleOutputs=off  AggregatedOutputs=off  SimulateUsing=Interpreted execution  OutOfRangeInputValueMessage=warning  NoRuleFiredMessage=warning  EmptyOutputFuzzySetMessage=warning
  Fuzzy Logic Controller2 : fuzblock/Fuzzy Logic  Controller  FIS='Untitled2.fis'  OutputSampleNumber=101  DataType=double  FuzzifiedInputs=off  RuleFiringStrengths=off  RuleOutputs=off  AggregatedOutputs=off  SimulateUsing=Interpreted execution  OutOfRangeInputValueMessage=warning  NoRuleFiredMessage=warning  EmptyOutputFuzzySetMessage=warning
  K1 : Gain  Gain=K0
  K2 : Gain  Gain=K0
  Kc : Gain  Gain=Kc
  Kc1 : Gain  Gain=-Kc
  Mux1 : Mux  Inputs=2
  Mux2 : Mux  Inputs=2
  Proportional Gain1 : Gain
  Proportional Gain2 : Gain
  Saturation1 : Saturate  UpperLimit=1  LowerLimit=-1
  Saturation2 : Saturate  UpperLimit=1  LowerLimit=-1
  Setpoint Weighting (Proportional)1 : Gain  DisableCoverage=on  Gain=b
  Setpoint Weighting (Proportional)2 : Gain  DisableCoverage=on  Gain=b
  Step : Step  Time=49  Before=1  After=0  SampleTime=Ts
  Step1 : Step  Time=49  Before=1  After=0  SampleTime=Ts
  Sum{1..2,5,7} (4 alike) : Sum  DisableCoverage=on  Inputs=+-
  Sum3 : Sum  Inputs=|++
  Sum6 : Sum  Inputs=|++
  kd1 : Gain  Gain=-Kd
  kd2 : Gain  Gain=-Kd
  ke1 : Gain  Gain=Ke
  ke2 : Gain  Gain=Ke
  Pitch : Outport  VectorParamsAs1DForOutWhenUnconnected=off
  Roll : Outport  Port=2  VectorParamsAs1DForOutWhenUnconnected=off
  wires:
  X_Ref/1 -> Sum1/1
  <dx>/1 -> Derivative Gain1/1
  <dy>/1 -> D 1/1
  Derivative Gain1/1 -> Sum3/2
  Proportional Gain1/1 -> Sum3/1
  Sum3/1 -> Kc/1
  <X>/1 -> Sum5/2, Sum1/2
  Sum5/1 -> Proportional Gain1/1
  K2/1 -> Setpoint Weighting (Proportional)1/1
  ke1/1 -> Mux1/1
  Saturation1/1 -> Fuzzy Logic Controller1/1
  <dx>1/1 -> kd1/1
  Mux1/1 -> Saturation1/1
  kd1/1 -> Mux1/2
  Setpoint Weighting (Proportional)1/1 -> Sum5/1
  Setpoint Weighting (Proportional)2/1 -> Sum7/1
  kd2/1 -> Mux2/2
  Mux2/1 -> Saturation2/1
  <dy>1/1 -> kd2/1
  Saturation2/1 -> Fuzzy Logic Controller2/1
  ke2/1 -> Mux2/1
  K1/1 -> Setpoint Weighting (Proportional)2/1
  Sum7/1 -> Proportional Gain2/1
  <Y>/1 -> Sum7/2, Sum2/2
  Proportional Gain2/1 -> Sum6/1
  D 1/1 -> Sum6/2
  Y_Ref/1 -> Sum2/1
  Sum6/1 -> Kc1/1
  Sum1/1 -> ke1/1
  Sum2/1 -> ke2/1
  Step/1 -> Discrete-Time Integrator4/2
  Fuzzy Logic Controller1/1 -> Discrete-Time Integrator4/1
  Discrete-Time Integrator4/1 -> K2/1
  Step1/1 -> Discrete-Time Integrator1/2
  Fuzzy Logic Controller2/1 -> Discrete-Time Integrator1/1
  Discrete-Time Integrator1/1 -> K1/1
  Kc/1 -> Pitch/1
  Kc1/1 -> Roll/1

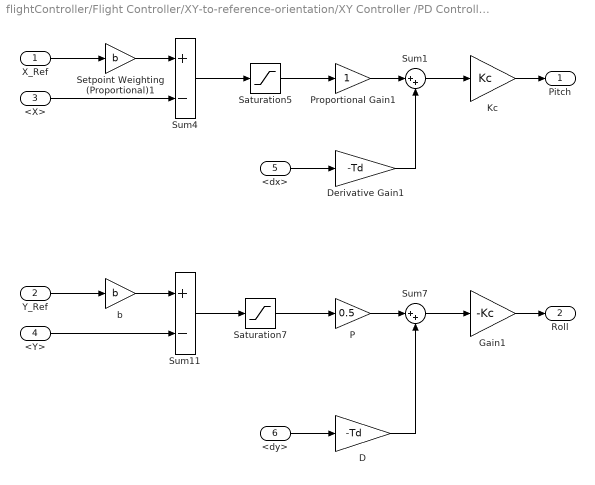
== system flightController/Flight Controller/XY-to-reference-orientation/XY Controller /PD Controller  ==
  X_Ref : Inport
  Y_Ref : Inport  Port=2
  <X> : Inport  Port=3
  <Y> : Inport  Port=4
  <dx> : Inport  Port=5
  <dy> : Inport  Port=6
  D : Gain  Gain=-Td
  Derivative Gain1 : Gain  DisableCoverage=on  Gain=-Td
  Gain1 : Gain  Gain=-Kc
  Kc : Gain  Gain=Kc
  P : Gain  Gain=0.5
  Proportional Gain1 : Gain
  Saturation5 : Saturate  UpperLimit=3  LowerLimit=-3  OutDataTypeStr=single
  Saturation7 : Saturate  UpperLimit=3  LowerLimit=-3  OutDataTypeStr=single
  Setpoint Weighting (Proportional)1 : Gain  DisableCoverage=on  Gain=b
  Sum1 : Sum  Inputs=|++
  Sum11 : Sum  DisableCoverage=on  Inputs=+-
  Sum4 : Sum  DisableCoverage=on  Inputs=+-
  Sum7 : Sum  Inputs=|++
  b : Gain  Gain=b
  Pitch : Outport  OutDataTypeStr=single  VectorParamsAs1DForOutWhenUnconnected=off
  Roll : Outport  Port=2  OutDataTypeStr=single  VectorParamsAs1DForOutWhenUnconnected=off
  wires:
  D/1 -> Sum7/2
  Derivative Gain1/1 -> Sum1/2
  Proportional Gain1/1 -> Sum1/1
  Sum1/1 -> Kc/1
  Sum4/1 -> Saturation5/1
  X_Ref/1 -> Setpoint Weighting (Proportional)1/1
  Saturation5/1 -> Proportional Gain1/1
  P/1 -> Sum7/1
  Saturation7/1 -> P/1
  b/1 -> Sum11/1
  Sum7/1 -> Gain1/1
  <X>/1 -> Sum4/2
  Y_Ref/1 -> b/1
  Setpoint Weighting (Proportional)1/1 -> Sum4/1
  Sum11/1 -> Saturation7/1
  <dy>/1 -> D/1
  <dx>/1 -> Derivative Gain1/1
  <Y>/1 -> Sum11/2
  Kc/1 -> Pitch/1
  Gain1/1 -> Roll/1

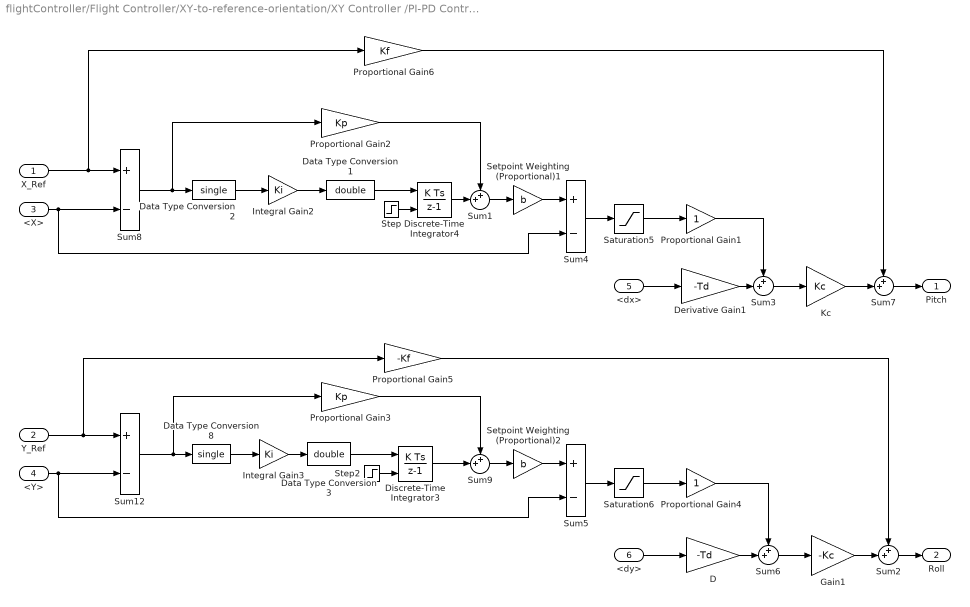
== system flightController/Flight Controller/XY-to-reference-orientation/XY Controller /PI-PD Controller  ==
  X_Ref : Inport
  Y_Ref : Inport  Port=2
  <X> : Inport  Port=3
  <Y> : Inport  Port=4
  <dx> : Inport  Port=5
  <dy> : Inport  Port=6
  D : Gain  Gain=-Td
  Data Type Conversion1 : DataTypeConversion  OutDataTypeStr=double  SaturateOnIntegerOverflow=off  RndMeth=Floor
  Data Type Conversion2 : DataTypeConversion  OutDataTypeStr=single  SaturateOnIntegerOverflow=off  RndMeth=Floor
  Data Type Conversion3 : DataTypeConversion  OutDataTypeStr=double  SaturateOnIntegerOverflow=off  RndMeth=Floor
  Data Type Conversion8 : DataTypeConversion  OutDataTypeStr=single  SaturateOnIntegerOverflow=off  RndMeth=Floor
  Derivative Gain1 : Gain  DisableCoverage=on  Gain=-Td
  Discrete-Time Integrator3 : DiscreteIntegrator  ExternalReset=falling  SampleTime=Ts  ICPrevOutput=DiscIntNeverNeededParam  ICPrevScaledInput=DiscIntNeverNeededParam
  Discrete-Time Integrator4 : DiscreteIntegrator  ExternalReset=falling  SampleTime=Ts  ICPrevOutput=DiscIntNeverNeededParam  ICPrevScaledInput=DiscIntNeverNeededParam
  Gain1 : Gain  Gain=-Kc
  Integral Gain2 : Gain  DisableCoverage=on  Gain=Ki
  Integral Gain3 : Gain  DisableCoverage=on  Gain=Ki
  Kc : Gain  Gain=Kc
  Proportional Gain1 : Gain
  Proportional Gain2 : Gain  Gain=Kp
  Proportional Gain3 : Gain  Gain=Kp
  Proportional Gain4 : Gain
  Proportional Gain5 : Gain  Gain=-Kf
  Proportional Gain6 : Gain  Gain=Kf
  Saturation5 : Saturate  UpperLimit=3  LowerLimit=-3  OutDataTypeStr=single
  Saturation6 : Saturate  UpperLimit=3  LowerLimit=-3  OutDataTypeStr=single
  Setpoint Weighting (Proportional)1 : Gain  DisableCoverage=on  Gain=b
  Setpoint Weighting (Proportional)2 : Gain  DisableCoverage=on  Gain=b
  Step : Step  Time=49  Before=1  After=0  SampleTime=Ts
  Step2 : Step  Time=49  Before=1  After=0  SampleTime=Ts
  Sum{1..3,6..7,9} (6 alike) : Sum  Inputs=++|
  Sum{4..5,8,12} (4 alike) : Sum  DisableCoverage=on  Inputs=+-
  Pitch : Outport  OutDataTypeStr=single  VectorParamsAs1DForOutWhenUnconnected=off
  Roll : Outport  Port=2  OutDataTypeStr=single  VectorParamsAs1DForOutWhenUnconnected=off
  wires:
  Proportional Gain4/1 -> Sum6/1
  D/1 -> Sum6/2
  Sum5/1 -> Saturation6/1
  Sum9/1 -> Setpoint Weighting (Proportional)2/1
  Saturation6/1 -> Proportional Gain4/1
  Setpoint Weighting (Proportional)2/1 -> Sum5/1
  Step2/1 -> Discrete-Time Integrator3/2
  Step/1 -> Discrete-Time Integrator4/2
  Proportional Gain3/1 -> Sum9/1
  Data Type Conversion3/1 -> Discrete-Time Integrator3/1
  Y_Ref/1 -> Proportional Gain5/1, Sum12/1
  Integral Gain3/1 -> Data Type Conversion3/1
  Discrete-Time Integrator3/1 -> Sum9/2
  Data Type Conversion8/1 -> Integral Gain3/1
  Sum12/1 -> Proportional Gain3/1, Data Type Conversion8/1
  Sum8/1 -> Proportional Gain2/1, Data Type Conversion2/1
  Data Type Conversion2/1 -> Integral Gain2/1
  Discrete-Time Integrator4/1 -> Sum1/2
  Integral Gain2/1 -> Data Type Conversion1/1
  Data Type Conversion1/1 -> Discrete-Time Integrator4/1
  Proportional Gain2/1 -> Sum1/1
  Kc/1 -> Sum7/2
  Gain1/1 -> Sum2/2
  <dx>/1 -> Derivative Gain1/1
  <dy>/1 -> D/1
  Derivative Gain1/1 -> Sum3/2
  Proportional Gain1/1 -> Sum3/1
  Setpoint Weighting (Proportional)1/1 -> Sum4/1
  Sum3/1 -> Kc/1
  <X>/1 -> Sum4/2, Sum8/2
  Sum6/1 -> Gain1/1
  <Y>/1 -> Sum5/2, Sum12/2
  Saturation5/1 -> Proportional Gain1/1
  Sum1/1 -> Setpoint Weighting (Proportional)1/1
  Sum4/1 -> Saturation5/1
  Proportional Gain5/1 -> Sum2/1
  Proportional Gain6/1 -> Sum7/1
  X_Ref/1 -> Sum8/1, Proportional Gain6/1
  Sum7/1 -> Pitch/1
  Sum2/1 -> Roll/1
